simulink model "Ampel"  (R2016a)
settings: Solver=FixedStepAuto  StartTime=0.0  StopTime=100.0  FixedStep=0.1  MaxStep=1e-2  RelTol=1e-3
model workspace (MAT data in the model file):
  DUR_AMBER = Simulink.Parameter
  DUR_AMBER.Value = 3
  DUR_AMBER.DataType = 'auto'
  DUR_AMBER.DocUnits = 'sec'
  DUR_AMBER.Dimensions = [1 1]
  DUR_GREEN = Simulink.Parameter
  DUR_GREEN.Value = 14
  DUR_GREEN.DataType = 'auto'
  DUR_GREEN.DocUnits = 'sec'
  DUR_GREEN.Dimensions = [1 1]
  DUR_RED = Simulink.Parameter
  DUR_RED.Value = 10
  DUR_RED.DataType = 'auto'
  DUR_RED.DocUnits = 'sec'
  DUR_RED.Dimensions = [1 1]
  DUR_REDAMBER = Simulink.Parameter
  DUR_REDAMBER.Value = 2
  DUR_REDAMBER.DataType = 'auto'
  DUR_REDAMBER.DocUnits = 'sec'
  DUR_REDAMBER.Dimensions = [1 1]
libraries: simulink x6, sldrtlib x1
settings Model: Creator=Dominik  LastModifiedBy=Dominik
settings GRTTargetCC: GeneratePreprocessorConditionals=Use local settings

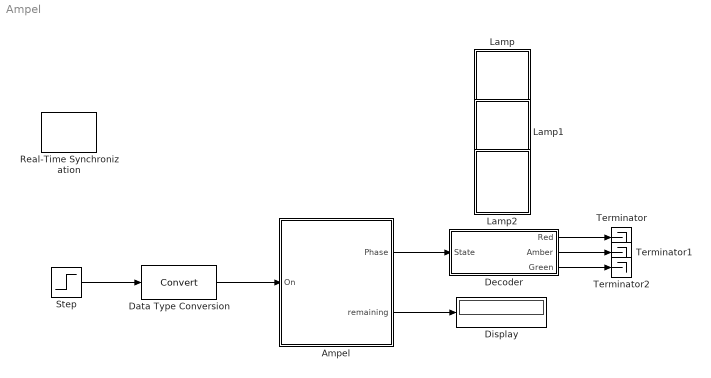
== system Ampel ==
  Ampel : Subsystem
  Data Type Conversion : DataTypeConversion
  Decoder : Subsystem
  Display : Display
  Lamp : Subsystem  DialogController=hmiCreateDDGDialog  IsWebBlock=on  mask(MWDashboardBlock){webBlockId=6ca87ed8-de92-47fd-b00b-4917f35fc017, webBlockType=lamp, ShowInLibBrowser=on, ShowInitialText=on, HMISrcModelName=Ampel}
      mask prompts: webBlockType "WebBlock Type"; HMISrcModelName "Source Model"
      mask Help: helpview([docroot '/mapfiles/simulink.map'], 'hmi_lamp')
      mask Display:
      | if strcmp(get_param(bdroot(gcb),'BlockDiagramType'), 'library')
      |     image([(matlabroot) '/toolbox/simulink/hmi/icons/Lamp.png']);
      | end
  Lamp1 : Subsystem  DialogController=hmiCreateDDGDialog  IsWebBlock=on  mask(MWDashboardBlock){webBlockId=43797351-e998-493e-9020-83e3557ff8af, webBlockType=lamp, ShowInLibBrowser=on, ShowInitialText=on, HMISrcModelName=Ampel}
      mask prompts: webBlockType "WebBlock Type"; HMISrcModelName "Source Model"
      mask Help: helpview([docroot '/mapfiles/simulink.map'], 'hmi_lamp')
      mask Display:
      | if strcmp(get_param(bdroot(gcb),'BlockDiagramType'), 'library')
      |     image([(matlabroot) '/toolbox/simulink/hmi/icons/Lamp.png']);
      | end
  Lamp2 : Subsystem  DialogController=hmiCreateDDGDialog  IsWebBlock=on  mask(MWDashboardBlock){webBlockId=9af26628-87b3-404d-806f-d9d7d1783e57, webBlockType=lamp, ShowInLibBrowser=on, ShowInitialText=on, HMISrcModelName=Ampel}
      mask prompts: webBlockType "WebBlock Type"; HMISrcModelName "Source Model"
      mask Help: helpview([docroot '/mapfiles/simulink.map'], 'hmi_lamp')
      mask Display:
      | if strcmp(get_param(bdroot(gcb),'BlockDiagramType'), 'library')
      |     image([(matlabroot) '/toolbox/simulink/hmi/icons/Lamp.png']);
      | end
  Real-Time Synchronization : sldrtlib/Real-Time Synchronization  SampleTime=0.1  MaxMissedTicks=10  ShowMissedTicks=off  YieldWhenWaiting=off
  Step : Step  Before=-1  SampleTime=0
  Terminator : Terminator
  Terminator1 : Terminator
  Terminator2 : Terminator
  wires:
  Step/1 -> Data Type Conversion/1
  Data Type Conversion/1 -> Ampel/1(On)
  Ampel/2(remaining) -> Display/1
  Ampel/1(Phase) -> Decoder/1(State)
  Decoder/1(Red) -> Terminator/1
  Decoder/2(Amber) -> Terminator1/1
  Decoder/3(Green) -> Terminator2/1

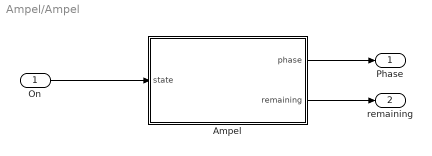
== system Ampel/Ampel ==
  On : Inport  OutDataTypeStr=boolean
  Ampel : Stateflow chart  TreatAsAtomicUnit=on
  Phase : Outport  OutDataTypeStr=Enum: TrafficLightPhase
  remaining : Outport  Port=2
  wires:
  Ampel/2(remaining) -> remaining/1
  Ampel/1(phase) -> Phase/1
  On/1 -> Ampel/1(state)

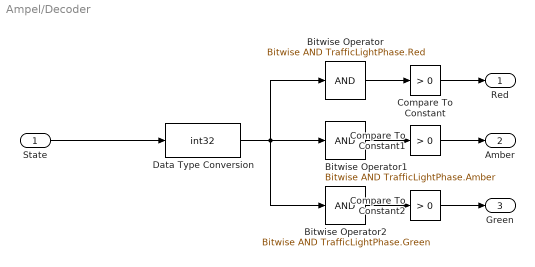
== system Ampel/Decoder ==
  State : Inport
  Bitwise Operator1 : simulink/Logic and Bit Operations/Bitwise Operator  logicop=AND  UseBitMask=on  BitMask=TrafficLightPhase.Amber  BitMaskRealWorld=Stored Integer
  Bitwise Operator2 : simulink/Logic and Bit Operations/Bitwise Operator  logicop=AND  UseBitMask=on  BitMask=TrafficLightPhase.Green  BitMaskRealWorld=Stored Integer
  Bitwise Operator : simulink/Logic and Bit Operations/Bitwise Operator  logicop=AND  UseBitMask=on  BitMask=TrafficLightPhase.Red  BitMaskRealWorld=Stored Integer
  Compare To Constant : simulink/Logic and Bit Operations/Compare To Constant  relop=>  const=0  OutDataTypeStr=boolean
  Compare To Constant1 : simulink/Logic and Bit Operations/Compare To Constant  relop=>  const=0  OutDataTypeStr=boolean
  Compare To Constant2 : simulink/Logic and Bit Operations/Compare To Constant  relop=>  const=0  OutDataTypeStr=boolean
  Data Type Conversion : DataTypeConversion  OutDataTypeStr=int32
  Red : Outport
  Amber : Outport  Port=2
  Green : Outport  Port=3
  wires:
  Bitwise Operator/1 -> Compare To Constant/1
  Bitwise Operator1/1 -> Compare To Constant1/1
  Bitwise Operator2/1 -> Compare To Constant2/1
  State/1 -> Data Type Conversion/1
  Data Type Conversion/1 -> Bitwise Operator/1, Bitwise Operator2/1, Bitwise Operator1/1
  Compare To Constant/1 -> Red/1
  Compare To Constant1/1 -> Amber/1
  Compare To Constant2/1 -> Green/1

== system Ampel/Lamp ==

== system Ampel/Lamp1 ==

== system Ampel/Lamp2 ==

== stateflow chart Ampel/Ampel ==
  state Off
    du: phase = TrafficLightPhase.Off;
  state On
    state RedAmber
      du:
      phase = TrafficLightPhase.RedAmber;
      remaining = DUR_REDAMBER - temporalCount(sec);
    state Red
      du:
      phase = TrafficLightPhase.Red;
      remaining = DUR_RED - temporalCount(sec);
    state Amber
      du:
      phase = TrafficLightPhase.Amber;
      remaining = DUR_AMBER - temporalCount(sec);
    state Green
      du:
      phase = TrafficLightPhase.Green;
      remaining = DUR_GREEN - temporalCount(sec);
    (default) -> Red
    Red -> RedAmber : after(DUR_RED, sec)
    Amber -> Red : after(DUR_AMBER, sec)
    RedAmber -> Green : after(DUR_REDAMBER, sec)
    Green -> Amber : after(DUR_GREEN, sec)
  (default) -> Off
  Off -> On : [state]
  On -> Off : [~state]
  data: phase output; remaining output; DUR_AMBER parameter; DUR_GREEN parameter; DUR_REDAMBER parameter; DUR_RED parameter; state input
